simulink library "ESTS_UOD_YawRateDeadZone"  (R2022a)
settings: Solver=VariableStepAuto  StartTime=0.0  StopTime=10.0  RelTol=1e-3
undefined symbols (not defined in the file or in its folder): ESTS_UOD_p_YawRateDeadZThd_degps
settings Model: Creator=blatak  LastModifiedBy=blatak

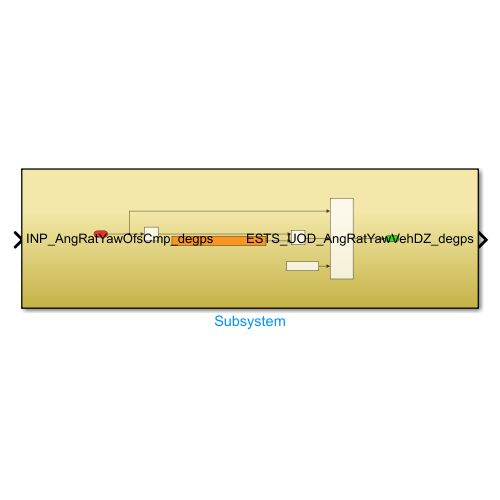
[thumbnail: Simulink's stored preview of the top-level diagram]
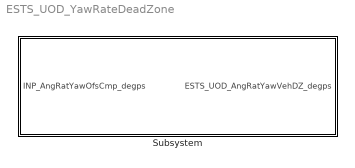
== system ESTS_UOD_YawRateDeadZone ==
  Subsystem : Subsystem

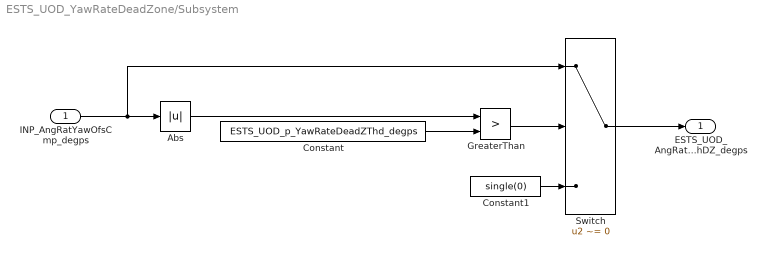
== system ESTS_UOD_YawRateDeadZone/Subsystem ==
  INP_AngRatYawOfsCmp_degps : Inport
  Abs : Abs  SaturateOnIntegerOverflow=off
  Constant : Constant  Value=ESTS_UOD_p_YawRateDeadZThd_degps
  Constant1 : Constant  Value=single(0)
  GreaterThan : RelationalOperator  Operator=>  OutDataTypeStr=boolean  RndMeth=Simplest  InputSameDT=off
  Switch : Switch  Criteria=u2 ~= 0  SaturateOnIntegerOverflow=off  InputSameDT=off
  ESTS_UOD_AngRatYawVehDZ_degps : Outport
  wires:
  GreaterThan/1 -> Switch/2
  Switch/1 -> ESTS_UOD_AngRatYawVehDZ_degps/1
  Constant/1 -> GreaterThan/2
  INP_AngRatYawOfsCmp_degps/1 -> Switch/1, Abs/1
  Constant1/1 -> Switch/3
  Abs/1 -> GreaterThan/1
